simulink model "groundStation001_th"  (R2020a)
settings: Solver=VariableStepAuto  StartTime=0.0  StopTime=simParams.duration.Value  FixedStep=1e-2  MaxStep=0.1*sqrt(simParams.lengthScaleFactor.Value)  RelTol=1e-3  AbsTol=1e-3
values from neighbouring files (symbols this model uses):
  D = sum(normalVecMat'.*relVelGnd',2)    [oceanForceFunct.m]
undefined symbols (not defined in the file or in its folder): gndStn, groundStation001, groundStation001_cl
libraries: vrlib x2, tethersMoment_cl x2, thrAttachPtKinematics_ul x2, dspstat3 x1, environment_cl x1, simulink x1, tether000_cl x1, bouyancyCalculator_ul x1, oceanForceCalculator_ul x1, sixDoFDynamicsEuler_ul x1
settings Model: SimulationMode=accelerator  Creator=Erin B  LastModifiedBy=jcreed2
settings DataIOCC: SaveOutput=off  DSMLogging=off  ReturnWorkspaceOutputs=off
settings DebuggingCC: ArithmeticOperatorsInVariantConditions=warning
settings SFSimCC: CustomCodeUndefinedFunction=UseInterfaceOnly

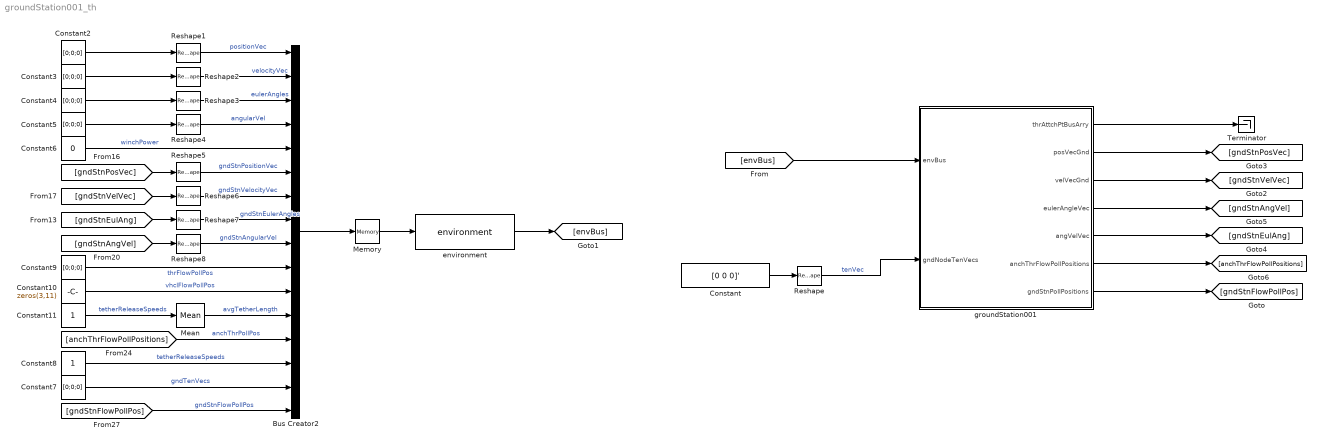
== system groundStation001_th ==
  Bus Creator2 : BusCreator  Inputs=16  OutDataTypeStr=Bus: plantBus  NonVirtualBus=on
  Constant : Constant  Value=[0 0 0]'
  Constant10 : Constant  Value=zeros(3,11)
  Constant11 : Constant
  Constant{2..5,7,9} (6 alike) : Constant  Value=[0;0;0]
  Constant6 : Constant  Value=0
  Constant8 : Constant
  Mean : dspstat3/Mean  run=off  InputProcessing=Columns as channels (frame based)  reset_popup=None  directionMode=Each column  dimension=1  roiEnable=off  roiType=Rectangles  roiPortion=Entire ROI  roiOutput=Individual statistics for each ROI  roiFlag=off  roundingMode=Floor  overflowMode=off  outputDataTypeStr=Inherit: Same as accumulator  outputMin=[]  outputMax=[]  outputLastDataTypeStr=Inherit: Same as accumulator
  Memory : Memory
  Reshape{,1..8} (9 alike) : Reshape  OutputDimensionality=Column vector (2-D)
  Terminator : Terminator
  environment : environment_cl/environment  SystemSampleTime=-1  Latency=0  AutoFrameSizeCalculation=off
  groundStation001 : Subsystem  AncestorBlock=groundStation001_cl/groundStation001  VariantControl=VSS_groundStation_groundStation001  mask{gs=gndStn, numNodes=2}
      mask prompts: gs "Ground Station"; numNodes "Number of anchor tether nodes"
      mask init:
      | groundStation001_init
  wires:
  groundStation001/1(thrAttchPtBusArry) -> Terminator/1
  Reshape/1 -> groundStation001/2(gndNodeTenVecs)  "tenVec"
  [envBus] -> groundStation001/1(envBus)
  Constant/1 -> Reshape/1
  groundStation001/2(posVecGnd) -> [gndStnPosVec]
  groundStation001/3(velVecGnd) -> [gndStnVelVec]
  groundStation001/4(eulerAngleVec) -> [gndStnAngVel]
  groundStation001/5(angVelVec) -> [gndStnEulAng]
  groundStation001/6(anchThrFlowPollPositions) -> [anchThrFlowPollPositions]
  groundStation001/7(gndStnPollPositions) -> [gndStnFlowPollPos]
  environment/1 -> [envBus]
  Memory/1 -> environment/1
  [gndStnEulAng] -> Reshape7/1
  Reshape5/1 -> Bus Creator2/6  "gndStnPositionVec"
  Constant5/1 -> Reshape4/1
  Reshape1/1 -> Bus Creator2/1  "positionVec"
  Bus Creator2/1 -> Memory/1
  Reshape2/1 -> Bus Creator2/2  "velocityVec"
  Reshape3/1 -> Bus Creator2/3  "eulerAngles"
  Reshape6/1 -> Bus Creator2/7  "gndStnVelocityVec"
  Constant3/1 -> Reshape2/1
  Constant4/1 -> Reshape3/1
  [gndStnFlowPollPos] -> Bus Creator2/16  "gndStnFlowPollPos"
  Constant8/1 -> Bus Creator2/14  "tetherReleaseSpeeds"
  [gndStnAngVel] -> Reshape8/1
  [gndStnVelVec] -> Reshape6/1
  Constant10/1 -> Bus Creator2/11  "vhclFlowPollPos"
  Constant9/1 -> Bus Creator2/10  "thrFlowPollPos"
  [anchThrFlowPollPositions] -> Bus Creator2/13  "anchThrPollPos"
  Reshape7/1 -> Bus Creator2/8  "gndStnEulerAngles"
  Reshape8/1 -> Bus Creator2/9  "gndStnAngularVel"
  [gndStnPosVec] -> Reshape5/1
  Constant6/1 -> Bus Creator2/5  "winchPower"
  Reshape4/1 -> Bus Creator2/4  "angularVel"
  Mean/1 -> Bus Creator2/12  "avgTetherLength"
  Constant7/1 -> Bus Creator2/15  "gndTenVecs"
  Constant2/1 -> Reshape1/1
  Constant11/1 -> Mean/1  "tetherReleaseSpeeds"

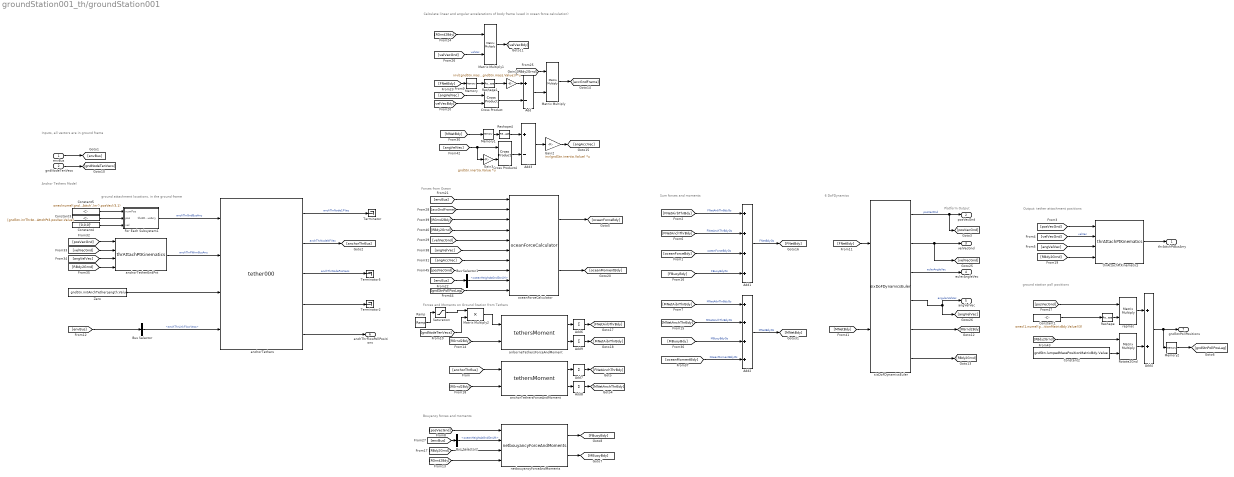
== system groundStation001_th/groundStation001 ==
  note: Forces from Ocean
  note: 6 DoFDynamics
  note: Sum forces and moments
  note: Inputs, all vectors are in ground frame
  note: Output: tether attachment positions
  note: Forces and Moments on Ground Station from Tethers
  note: Anchor Tethers Model
  note: Platform Output
  note: ground attachment locations, in the ground frame
  note: Calculate linear and angular accelerations of body frame
      | (used in ocean force calculation)
  note: Bouyancy forces and moments
  note: ground station poll positions
  envBus : Inport  OutDataTypeStr=Bus: envBus
  gndNodeTenVecs : Inport  Port=2
  Add : Sum  Inputs=+-
  Add1 : Sum  Inputs=++++
  Add2 : Sum  Inputs=++++
  Add3 : Sum  Inputs=+-
  Add4 : Sum
  Add{6..9} (4 alike) : Sum  Inputs=+  CollapseMode=Specified dimension  CollapseDim=2
  Bus Selector : BusSelector  OutputSignals=anchThrLinkFlowVecs
  Bus Selector1 : BusSelector  OutputSignals=oceanHeightAtGndStnLM
  Bus Selector2 : BusSelector  OutputSignals=oceanHeightAtGndStnLM
  Constant1 : Constant  Value=ones(1,numel(gndStn.lumpedMassPositionMatrixBdy.Value)/3)
  Constant2 : Constant  Value=gndStn.lumpedMassPositionMatrixBdy.Value
  Constant3 : Constant  Value=[gndStn.inrThrAttchPt1.posVec.Value,gndStn.inrThrAttchPt2.posVec.Value,gndStn.inrThrAttchPt3.posVec.Value]
  Constant4 : Constant  Value=[0,0,0]'
  Constant5 : Constant  Value=ones(numel(gndStn.struct('OCT.thrAttch','inr').posVec)/3,1)
  Cross Product : vrlib/Utilities/Cross Product
  Cross Product4 : vrlib/Utilities/Cross Product
  For Each Subsystem1 : Subsystem  TreatAsAtomicUnit=on
  Gain1 : Gain  Gain=inv([gndStn.mass.Value,0,0;0,gndStn.mass.Value,0;0,0,gndStn.mass.Value])  Multiplication=Matrix(K*u)
  Gain2 : Gain  Gain=inv(gndStn.inertia.Value)  Multiplication=Matrix(K*u)
  Gain3 : Gain  Gain=gndStn.inertia.Value  Multiplication=Matrix(K*u)
  Matrix Multiply : Product  Multiplication=Matrix(*)
  Matrix Multiply1 : Product  Multiplication=Matrix(*)
  Matrix Multiply2 : Product
  Memory : Memory
  Memory1 : Memory
  Memory2 : Memory  InitialCondition=gndStn.lumpedMassPositionMatrixBdy.Value
  Ramp : simulink/Sources/Ramp  slope=.0025  start=400  InitialOutput=0
  Reshape : Reshape  OutputDimensionality=Row vector (2-D)
  Reshape1 : Reshape  OutputDimensionality=Column vector (2-D)
  Reshape4 : Reshape  OutputDimensionality=Column vector (2-D)
  Rotate2Gnd : Product  Multiplication=Matrix(*)
  Saturation : Saturate
  Terminator : Terminator
  Terminator2 : Terminator
  Terminator5 : Terminator
  Zero : Constant  Value=gndStn.initAnchTetherLength.Value  OutDataTypeStr=Inherit: Inherit via back propagation
  airborneTethersForceAndMoment : tethersMoment_cl/tethersMoment  arms=gs.struct('OCT.thrAttch','kit')
  anchorTetherEndPnt : thrAttachPtKinematics_ul/thrAttachPtKinematics  atchPts=gs.struct('OCT.thrAttch','plt')
  anchorTethers : tether000_cl/tether000  VariantControl=VSS_tethers_tether000  LabelModeActiveChoice=twoNodeTether  numNodes=2  thrStructure=gs.anchThrs.struct('OCT.tether')  fluidDensity=env.water.density.Value  gravity=env.gravAccel.Value
  anchorTethersForceAndMoment : tethersMoment_cl/tethersMoment  arms=gs.struct('OCT.thrAttch','plt')
  netbouyancyForceAndMoments : bouyancyCalculator_ul/netbouyancyForceAndMoments  SystemSampleTime=-1  Latency=0  AutoFrameSizeCalculation=off
  oceanForceCalculator : oceanForceCalculator_ul/oceanForceCalculator  Cdx=gndStn.cdX.Value  Cdy=gndStn.cdY.Value  Cdz=gndStn.cdZ.Value  Cax=gndStn.aMX.Value  Cay=gndStn.aMY.Value  Caz=gndStn.aMZ.Value  V=gndStn.volume.Value/(numel(gndStn.lumpedMassPositionMatrixBdy.Value)/3)
  repmat : Product  Multiplication=Matrix(*)
  sixDoFDynamicsEuler : sixDoFDynamicsEuler_ul/sixDoFDynamicsEuler  VariantControl=(default)  M=gndStn.mass.Value  J=gndStn.inertia.Value  initPos=gndStn.initPosVecGnd.Value  initVel=gndStn.initVelVecBdy.Value  initEulAngs=gndStn.initEulAng.Value  initAngVel=gndStn.initAngVelVec.Value
  thrAttachPtKinematics : thrAttachPtKinematics_ul/thrAttachPtKinematics  atchPts=gs.struct('OCT.thrAttch','kit')
  thrAttchPtBusArry : Outport  VectorParamsAs1DForOutWhenUnconnected=off
  posVecGnd : Outport  Port=2  VectorParamsAs1DForOutWhenUnconnected=off
  velVecGnd : Outport  Port=3  VectorParamsAs1DForOutWhenUnconnected=off
  eulerAngleVec : Outport  Port=4  VectorParamsAs1DForOutWhenUnconnected=off
  angVelVec : Outport  Port=5  VectorParamsAs1DForOutWhenUnconnected=off
  anchThrFlowPollPositions : Outport  Port=6  VectorParamsAs1DForOutWhenUnconnected=off
  gndStnPollPositions : Outport  Port=7  VectorParamsAs1DForOutWhenUnconnected=off
  wires:
  Saturation/1 -> Matrix Multiply2/1
  Ramp/1 -> Saturation/1
  Matrix Multiply2/1 -> airborneTethersForceAndMoment/1
  [gndNodeTenVecs] -> Matrix Multiply2/2
  [gndStnPollPosLag] -> oceanForceCalculator/10
  Memory2/1 -> [gndStnPollPosLag]
  Add4/1 -> gndStnPollPositions/1, Memory2/1
  [envBus] -> Bus Selector2/1
  Bus Selector2/1 -> netbouyancyForceAndMoments/2  "<oceanHeightAtGndStnLM>"
  Bus Selector1/1 -> oceanForceCalculator/9  "<oceanHeightAtGndStnLM>"
  [envBus] -> Bus Selector1/1
  anchorTethers/5 -> anchThrFlowPollPositions/1
  Constant3/1 -> For Each Subsystem1/2(pos)
  Constant4/1 -> For Each Subsystem1/3(vel)
  Constant5/1 -> For Each Subsystem1/1(numPos)
  [posVecGnd] -> oceanForceCalculator/8
  Memory1/1 -> Reshape4/1
  Memory/1 -> Reshape1/1
  Reshape/1 -> repmat/2
  Bus Selector/1 -> anchorTethers/4  "<anchThrLinkFlowVecs>"
  [envBus] -> Bus Selector/1
  For Each Subsystem1/1(thrAttchPtBusArry) -> anchorTethers/1  "anchThrGndBusArry"
  Zero/1 -> anchorTethers/3
  [posVecGnd] -> repmat/1
  Constant1/1 -> Reshape/1
  Constant2/1 -> Rotate2Gnd/2
  Rotate2Gnd/1 -> Add4/2
  [RBdy2Grnd] -> Rotate2Gnd/1
  repmat/1 -> Add4/1
  [RBdy2Grnd] -> oceanForceCalculator/4
  [RGrnd2Bdy] -> oceanForceCalculator/3
  [angVelVec] -> oceanForceCalculator/6
  [angAccVec] -> oceanForceCalculator/7
  [velVecGnd] -> oceanForceCalculator/5
  [oceanMomentBdy] -> Add2/4  "OceanMomentBdyGs"
  oceanForceCalculator/2 -> [oceanMomentBdy]
  [accGndFrame] -> oceanForceCalculator/2
  Gain2/1 -> [angAccVec]
  Gain3/1 -> Cross Product4/2
  Reshape4/1 -> Add3/1
  Add3/1 -> Gain2/1
  Cross Product4/1 -> Add3/2
  [MNetBdy] -> Memory1/1
  [angVelVec] -> Gain3/1, Cross Product4/1
  Matrix Multiply/1 -> [accGndFrame]
  Matrix Multiply1/1 -> [velVecBdy]
  [RGrnd2Bdy] -> Matrix Multiply1/1
  [velVecGnd] -> Matrix Multiply1/2  "velVec"
  [RBdy2Grnd] -> Matrix Multiply/1
  Add/1 -> Matrix Multiply/2
  Gain1/1 -> Add/1
  Reshape1/1 -> Gain1/1
  [FNetBdy] -> Memory/1
  Cross Product/1 -> Add/2
  [velVecBdy] -> Cross Product/2
  [angVelVec] -> Cross Product/1
  [RBdy2Grnd] -> netbouyancyForceAndMoments/3
  [RGrnd2Bdy] -> netbouyancyForceAndMoments/4
  netbouyancyForceAndMoments/1 -> [FBuoyBdy]
  netbouyancyForceAndMoments/2 -> [MBuoyBdy]
  anchorTethers/4 -> Terminator2/1
  sixDoFDynamicsEuler/6 -> [RBdy2Grnd]
  sixDoFDynamicsEuler/5 -> [RGrnd2Bdy]
  sixDoFDynamicsEuler/4 -> angVelVec/1, [angVelVec]  "angularVelVec"
  sixDoFDynamicsEuler/2 -> velVecGnd/1, [velVecGnd]
  oceanForceCalculator/1 -> [oceanForceBdy]
  [envBus] -> oceanForceCalculator/1
  [FBuoyBdy] -> Add1/4  "FBuoyBdyGs"
  [MNetAnchThrBdy] -> Add2/2  "MNetAnchThrBdyGs"
  [MNetAibrThrBdy] -> Add2/1  "MNetAibrThrBdyGs"
  [FNetAnchThrBdy] -> Add1/2  "FNetAnchThrBdyGs"
  [FNetAirbThrBdy] -> Add1/1  "FNetAirbThrBdyGs"
  [anchorThrBus] -> anchorTethersForceAndMoment/1
  airborneTethersForceAndMoment/2 -> Add9/1
  airborneTethersForceAndMoment/1 -> Add6/1
  Add6/1 -> [FNetAirbThrBdy]
  Add9/1 -> [MNetAibrThrBdy]
  [RGrnd2Bdy] -> airborneTethersForceAndMoment/2
  [oceanForceBdy] -> Add1/3  "oceanForceBdyGs"
  envBus/1 -> [envBus]
  Add2/1 -> [MNetBdy]  "MNetBdyGs"
  gndNodeTenVecs/1 -> [gndNodeTenVecs]
  thrAttachPtKinematics/1 -> thrAttchPtBusArry/1
  [posVecGnd] -> thrAttachPtKinematics/1
  [angVelVec] -> thrAttachPtKinematics/3
  [RBdy2Grnd] -> thrAttachPtKinematics/4
  [velVecGnd] -> thrAttachPtKinematics/2  "velVec"
  Add8/1 -> [MNetAnchThrBdy]
  Add7/1 -> [FNetAnchThrBdy]
  anchorTethersForceAndMoment/2 -> Add8/1
  anchorTethersForceAndMoment/1 -> Add7/1
  [velVecGnd] -> anchorTetherEndPnt/2
  [RBdy2Grnd] -> anchorTetherEndPnt/4
  [angVelVec] -> anchorTetherEndPnt/3
  [posVecGnd] -> anchorTetherEndPnt/1
  [posVecGnd] -> netbouyancyForceAndMoments/1
  [MNetBdy] -> sixDoFDynamicsEuler/2
  [RGrnd2Bdy] -> anchorTethersForceAndMoment/2
  sixDoFDynamicsEuler/1 -> posVecGnd/1, [posVecGnd]  "posVecGnd"
  anchorTetherEndPnt/1 -> anchorTethers/2  "anchThrPltfrmBusArry"
  sixDoFDynamicsEuler/3 -> eulerAngleVec/1  "eulerAngleVec"
  anchorTethers/1 -> Terminator/1  "anchThrNode1FVec"
  anchorTethers/2 -> [anchorThrBus]  "anchThrNodeNFVec"
  Add1/1 -> [FNetBdy]  "FNetBdyGs"
  anchorTethers/3 -> Terminator5/1  "anchThrNodePosVecs"
  [FNetBdy] -> sixDoFDynamicsEuler/1
  [MBuoyBdy] -> Add2/3  "MBuoyBdyGs"

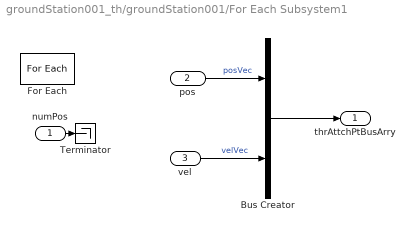
== system groundStation001_th/groundStation001/For Each Subsystem1 ==
  numPos : Inport  Partition=on  PartitionDimension=1  PartitionWidth=1  PartitionOffset=0
  pos : Inport  Port=2  Partition=on  PartitionDimension=2  PartitionWidth=1  PartitionOffset=0
  vel : Inport  Port=3
  Bus Creator : BusCreator  Inputs=2  OutDataTypeStr=Bus: thrAttachPtKinematicsBus  NonVirtualBus=on
  For Each : ForEach  DisableCoverage=on
  Terminator : Terminator
  thrAttchPtBusArry : Outport  ConcatenationDimension=1  VectorParamsAs1DForOutWhenUnconnected=off
  wires:
  numPos/1 -> Terminator/1
  vel/1 -> Bus Creator/2  "velVec"
  Bus Creator/1 -> thrAttchPtBusArry/1
  pos/1 -> Bus Creator/1  "posVec"
